simulink model "model_compatible"  (Simulink 7.5)
(part 2 of 2)

  bus83 : powerlib/Measurements/Load Flow Bus  LConnTagsString=a  Phases=single  Connectors=on one side  ID=bus83  Vbase=220000  Vref=1  Vangle=0  VLF=1  VLFb=1  VLFc=1  angleLF=0  angleLFb=0  angleLFc=0
      settings: AttributesFormatString=|
      | %<ID>
      | %<Vbase>V
      | %<VLF>pu
      | %<angleLF>deg.
      | %<Name>
  bus84 : powerlib/Measurements/Load Flow Bus  LConnTagsString=a  Phases=single  Connectors=on one side  ID=bus84  Vbase=220000  Vref=1  Vangle=0  VLF=1  VLFb=1  VLFc=1  angleLF=0  angleLFb=0  angleLFc=0
      settings: AttributesFormatString=|
      | %<ID>
      | %<Vbase>V
      | %<VLF>pu
      | %<angleLF>deg.
      | %<Name>
  bus85 : powerlib/Measurements/Load Flow Bus  LConnTagsString=a  Phases=single  Connectors=on one side  ID=bus85  Vbase=220000  Vref=1  Vangle=0  VLF=1  VLFb=1  VLFc=1  angleLF=0  angleLFb=0  angleLFc=0
      settings: AttributesFormatString=|
      | %<ID>
      | %<Vbase>V
      | %<VLF>pu
      | %<angleLF>deg.
      | %<Name>
  bus86 : powerlib/Measurements/Load Flow Bus  LConnTagsString=a  Phases=single  Connectors=on one side  ID=bus86  Vbase=220000  Vref=1  Vangle=0  VLF=1  VLFb=1  VLFc=1  angleLF=0  angleLFb=0  angleLFc=0
      settings: AttributesFormatString=|
      | %<ID>
      | %<Vbase>V
      | %<VLF>pu
      | %<angleLF>deg.
      | %<Name>
  bus87 : powerlib/Measurements/Load Flow Bus  LConnTagsString=a  Phases=single  Connectors=on one side  ID=bus87  Vbase=220000  Vref=1  Vangle=0  VLF=1  VLFb=1  VLFc=1  angleLF=0  angleLFb=0  angleLFc=0
      settings: AttributesFormatString=|
      | %<ID>
      | %<Vbase>V
      | %<VLF>pu
      | %<angleLF>deg.
      | %<Name>
  bus88 : powerlib/Measurements/Load Flow Bus  LConnTagsString=a  Phases=single  Connectors=on one side  ID=bus88  Vbase=220000  Vref=1  Vangle=0  VLF=1  VLFb=1  VLFc=1  angleLF=0  angleLFb=0  angleLFc=0
      settings: AttributesFormatString=|
      | %<ID>
      | %<Vbase>V
      | %<VLF>pu
      | %<angleLF>deg.
      | %<Name>
  bus89 : powerlib/Measurements/Load Flow Bus  LConnTagsString=a  Phases=single  Connectors=on one side  ID=bus89  Vbase=220000  Vref=1  Vangle=0  VLF=1  VLFb=1  VLFc=1  angleLF=0  angleLFb=0  angleLFc=0
      settings: AttributesFormatString=|
      | %<ID>
      | %<Vbase>V
      | %<VLF>pu
      | %<angleLF>deg.
      | %<Name>
  bus9 : powerlib/Measurements/Load Flow Bus  LConnTagsString=a  Phases=single  Connectors=on one side  ID=bus9  Vbase=220000  Vref=1  Vangle=0  VLF=1  VLFb=1  VLFc=1  angleLF=0  angleLFb=0  angleLFc=0
      settings: AttributesFormatString=|
      | %<ID>
      | %<Vbase>V
      | %<VLF>pu
      | %<angleLF>deg.
      | %<Name>
  bus90 : powerlib/Measurements/Load Flow Bus  LConnTagsString=a  Phases=single  Connectors=on one side  ID=bus90  Vbase=220000  Vref=1  Vangle=0  VLF=1  VLFb=1  VLFc=1  angleLF=0  angleLFb=0  angleLFc=0
      settings: AttributesFormatString=|
      | %<ID>
      | %<Vbase>V
      | %<VLF>pu
      | %<angleLF>deg.
      | %<Name>
  bus91 : powerlib/Measurements/Load Flow Bus  LConnTagsString=a  Phases=single  Connectors=on one side  ID=bus91  Vbase=220000  Vref=1  Vangle=0  VLF=1  VLFb=1  VLFc=1  angleLF=0  angleLFb=0  angleLFc=0
      settings: AttributesFormatString=|
      | %<ID>
      | %<Vbase>V
      | %<VLF>pu
      | %<angleLF>deg.
      | %<Name>
  bus92 : powerlib/Measurements/Load Flow Bus  LConnTagsString=a  Phases=single  Connectors=on one side  ID=bus92  Vbase=220000  Vref=1  Vangle=0  VLF=1  VLFb=1  VLFc=1  angleLF=0  angleLFb=0  angleLFc=0
      settings: AttributesFormatString=|
      | %<ID>
      | %<Vbase>V
      | %<VLF>pu
      | %<angleLF>deg.
      | %<Name>
  bus93 : powerlib/Measurements/Load Flow Bus  LConnTagsString=a  Phases=single  Connectors=on one side  ID=bus93  Vbase=220000  Vref=1  Vangle=0  VLF=1  VLFb=1  VLFc=1  angleLF=0  angleLFb=0  angleLFc=0
      settings: AttributesFormatString=|
      | %<ID>
      | %<Vbase>V
      | %<VLF>pu
      | %<angleLF>deg.
      | %<Name>
  bus94 : powerlib/Measurements/Load Flow Bus  LConnTagsString=a  Phases=single  Connectors=on one side  ID=bus94  Vbase=220000  Vref=1  Vangle=0  VLF=1  VLFb=1  VLFc=1  angleLF=0  angleLFb=0  angleLFc=0
      settings: AttributesFormatString=|
      | %<ID>
      | %<Vbase>V
      | %<VLF>pu
      | %<angleLF>deg.
      | %<Name>
  bus95 : powerlib/Measurements/Load Flow Bus  LConnTagsString=a  Phases=single  Connectors=on one side  ID=bus95  Vbase=220000  Vref=1  Vangle=0  VLF=1  VLFb=1  VLFc=1  angleLF=0  angleLFb=0  angleLFc=0
      settings: AttributesFormatString=|
      | %<ID>
      | %<Vbase>V
      | %<VLF>pu
      | %<angleLF>deg.
      | %<Name>
  bus96 : powerlib/Measurements/Load Flow Bus  LConnTagsString=a  Phases=single  Connectors=on one side  ID=bus96  Vbase=220000  Vref=1  Vangle=0  VLF=1  VLFb=1  VLFc=1  angleLF=0  angleLFb=0  angleLFc=0
      settings: AttributesFormatString=|
      | %<ID>
      | %<Vbase>V
      | %<VLF>pu
      | %<angleLF>deg.
      | %<Name>
  bus97 : powerlib/Measurements/Load Flow Bus  LConnTagsString=a  Phases=single  Connectors=on one side  ID=bus97  Vbase=220000  Vref=1  Vangle=0  VLF=1  VLFb=1  VLFc=1  angleLF=0  angleLFb=0  angleLFc=0
      settings: AttributesFormatString=|
      | %<ID>
      | %<Vbase>V
      | %<VLF>pu
      | %<angleLF>deg.
      | %<Name>
  bus98 : powerlib/Measurements/Load Flow Bus  LConnTagsString=a  Phases=single  Connectors=on one side  ID=bus98  Vbase=220000  Vref=1  Vangle=0  VLF=1  VLFb=1  VLFc=1  angleLF=0  angleLFb=0  angleLFc=0
      settings: AttributesFormatString=|
      | %<ID>
      | %<Vbase>V
      | %<VLF>pu
      | %<angleLF>deg.
      | %<Name>
  bus99 : powerlib/Measurements/Load Flow Bus  LConnTagsString=a  Phases=single  Connectors=on one side  ID=bus99  Vbase=220000  Vref=1  Vangle=0  VLF=1  VLFb=1  VLFc=1  angleLF=0  angleLFb=0  angleLFc=0
      settings: AttributesFormatString=|
      | %<ID>
      | %<Vbase>V
      | %<VLF>pu
      | %<angleLF>deg.
      | %<Name>
  powergui : powerlib/powergui  Priority=1  SimulationMode=Phasor  SolverType=Tustin/Backward Euler (TBE)  SampleTime=50e-6  frequency=50  SPID=off  DisableSnubberDevices=off  DisableRonSwitches=off  DisableVfSwitches=off  SwTol=0  DisplayEquations=off  Interpol=off  ExternalGateDelay=off  methode=off  Ts=10  FunctionMessages=off  echomessages=off  HookPort=off  EnableUseOfTLC=off  x0status=blocks  frequencyindice=50  Pbase=3000e6  ErrMax=0.0001  Iterations=50  UnitsV=V  UnitsW=W  buscounter=0  RestoreLinks=warning  ResistiveCurrentMeasurement=off  Frange=[0:2:500]  Ylog=off  Xlog=on  ShowGrid=off  save=off  variable=ZData  structure=0  ZoomFFT=off  StartTime=0.0  cycles=1  DisplayStyle=1  fundamental=60  FreqAxis=off  MaxFrequency=1000  frequencyindicesteady=1  RmsSteady=1  display=off
  connections:
  T_174347010_220000_Centrale_Electrique_de_Oued_Sly/LConn1 -- _CN_174347010_220000_CN_173670736_220000/LConn1
  T_174347010_220000_Centrale_Electrique_de_Oued_Sly/LConn2 -- _CN_174347010_220000_CN_173670736_220000/LConn2
  _CN_174347010_220000_CN_173670736_220000/LConn3 -- T_174347010_220000_Centrale_Electrique_de_Oued_Sly/LConn3 -- bus1/LConn1
  _CN_174347010_220000_CN_173670736_220000/RConn1 -- T_173670736_220000_Poste_électrique_de_Khemis_Miliana/LConn1 -- _CN_375972637_220000_CN_173670736_220000/LConn1
  _CN_174347010_220000_CN_173670736_220000/RConn2 -- T_173670736_220000_Poste_électrique_de_Khemis_Miliana/LConn2 -- _CN_375972637_220000_CN_173670736_220000/LConn2
  _CN_174347010_220000_CN_173670736_220000/RConn3 -- T_173670736_220000_Poste_électrique_de_Khemis_Miliana/LConn3 -- _CN_375972637_220000_CN_173670736_220000/LConn3 -- bus2/LConn1
  _CN_177004931_220000_CN_173534563_220000/LConn1 -- T_177004931__Poste_électrique_de_Chefia/RConn1 -- _CN_177004931_220000_CN_177004925_220000/LConn1 -- L_177004931/LConn1
  _CN_177004931_220000_CN_173534563_220000/LConn2 -- T_177004931__Poste_électrique_de_Chefia/RConn2 -- _CN_177004931_220000_CN_177004925_220000/LConn2 -- L_177004931/LConn2
  _CN_177004931_220000_CN_173534563_220000/LConn3 -- T_177004931__Poste_électrique_de_Chefia/RConn3 -- _CN_177004931_220000_CN_177004925_220000/LConn3 -- L_177004931/LConn3 -- bus3/LConn1
  _CN_177004931_220000_CN_173534563_220000/RConn1 -- T_173534563_220000_/LConn1 -- _CN_173534563_220000_CN_177004925_220000/LConn1 -- _CN_173534563_220000_CN_176932212_220000/LConn1
  _CN_177004931_220000_CN_173534563_220000/RConn2 -- T_173534563_220000_/LConn2 -- _CN_173534563_220000_CN_177004925_220000/LConn2 -- _CN_173534563_220000_CN_176932212_220000/LConn2
  _CN_177004931_220000_CN_173534563_220000/RConn3 -- T_173534563_220000_/LConn3 -- _CN_173534563_220000_CN_177004925_220000/LConn3 -- _CN_173534563_220000_CN_176932212_220000/LConn3 -- bus4/LConn1
  _CN_177004931_220000_CN_177004925_220000/RConn1 -- T_177004925__/LConn1 -- _CN_173534563_220000_CN_177004925_220000/RConn1
  _CN_177004931_220000_CN_177004925_220000/RConn2 -- T_177004925__/LConn2 -- _CN_173534563_220000_CN_177004925_220000/RConn2
  _CN_177004931_220000_CN_177004925_220000/RConn3 -- T_177004925__/LConn3 -- _CN_173534563_220000_CN_177004925_220000/RConn3 -- bus5/LConn1
  _CN_295277014_220000_CN_174419698_220000/LConn1 -- T_295277014_220000_/LConn1 -- _CN_295277014_220000_CN_176684982_220000/LConn1
  _CN_295277014_220000_CN_174419698_220000/LConn2 -- T_295277014_220000_/LConn2 -- _CN_295277014_220000_CN_176684982_220000/LConn2
  _CN_295277014_220000_CN_174419698_220000/LConn3 -- T_295277014_220000_/LConn3 -- _CN_295277014_220000_CN_176684982_220000/LConn3 -- bus6/LConn1
  _CN_295277014_220000_CN_174419698_220000/RConn1 -- T_174419698__/LConn1 -- _CN_174512806_220000_CN_174419698_220000/LConn1 -- _CN_174512286_220000_CN_174419698_220000/LConn1
  _CN_295277014_220000_CN_174419698_220000/RConn2 -- T_174419698__/LConn2 -- _CN_174512806_220000_CN_174419698_220000/LConn2 -- _CN_174512286_220000_CN_174419698_220000/LConn2
  _CN_295277014_220000_CN_174419698_220000/RConn3 -- T_174419698__/LConn3 -- _CN_174512806_220000_CN_174419698_220000/LConn3 -- bus7/LConn1 -- _CN_174512286_220000_CN_174419698_220000/LConn3
  _CN_295277014_220000_CN_176684982_220000/RConn1 -- T_176684982_220000_/LConn1 -- _CN_176684982_220000_CN_226914785_220000/LConn1 -- _CN_176684982_220000_CN_175343993_220000/LConn1
  _CN_295277014_220000_CN_176684982_220000/RConn2 -- T_176684982_220000_/LConn2 -- _CN_176684982_220000_CN_226914785_220000/LConn2 -- _CN_176684982_220000_CN_175343993_220000/LConn2
  _CN_295277014_220000_CN_176684982_220000/RConn3 -- T_176684982_220000_/LConn3 -- _CN_176684982_220000_CN_226914785_220000/LConn3 -- _CN_176684982_220000_CN_175343993_220000/LConn3 -- bus8/LConn1
  _CN_218114438_220000_CN_217976993_220000/LConn1 -- T_218114438__Centrale_Electrique/LConn1 -- _CN_218114438_220000_CN_364421786_220000/LConn1
  _CN_218114438_220000_CN_217976993_220000/LConn2 -- T_218114438__Centrale_Electrique/LConn2 -- _CN_218114438_220000_CN_364421786_220000/LConn2
  _CN_218114438_220000_CN_217976993_220000/LConn3 -- T_218114438__Centrale_Electrique/LConn3 -- _CN_218114438_220000_CN_364421786_220000/LConn3 -- bus9/LConn1
  _CN_218114438_220000_CN_217976993_220000/RConn1 -- T_217976993__/LConn1 -- _CN_217970970_220000_CN_217976993_220000/LConn1 -- _CN_217976993_220000_CN_217926709_220000/LConn1
  _CN_218114438_220000_CN_217976993_220000/RConn2 -- T_217976993__/LConn2 -- _CN_217970970_220000_CN_217976993_220000/LConn2 -- _CN_217976993_220000_CN_217926709_220000/LConn2
  _CN_218114438_220000_CN_217976993_220000/RConn3 -- T_217976993__/LConn3 -- _CN_217970970_220000_CN_217976993_220000/LConn3 -- _CN_217976993_220000_CN_217926709_220000/LConn3 -- bus10/LConn1
  _CN_218114438_220000_CN_364421786_220000/RConn1 -- G_364421786_/RConn1 -- _CN_217941443_220000_CN_364421786_220000/LConn1
  _CN_218114438_220000_CN_364421786_220000/RConn2 -- G_364421786_/RConn2 -- _CN_217941443_220000_CN_364421786_220000/LConn2
  _CN_218114438_220000_CN_364421786_220000/RConn3 -- G_364421786_/RConn3 -- _CN_217941443_220000_CN_364421786_220000/LConn3 -- bus11/LConn1
  _CN_93235592_220000_CN_143736898_220000/LConn1 -- T_93235592_220000_SONELGAZ/LConn1 -- _CN_93235592_220000_CN_380986745_220000/LConn1
  _CN_93235592_220000_CN_143736898_220000/LConn2 -- T_93235592_220000_SONELGAZ/LConn2 -- _CN_93235592_220000_CN_380986745_220000/LConn2
  _CN_93235592_220000_CN_143736898_220000/LConn3 -- T_93235592_220000_SONELGAZ/LConn3 -- _CN_93235592_220000_CN_380986745_220000/LConn3 -- bus12/LConn1
  _CN_93235592_220000_CN_143736898_220000/RConn1 -- T_143736898__/LConn1 -- _CN_143736898_220000_CN_173808767_220000/LConn1 -- _CN_143736898_220000_CN_380986745_220000/LConn1
  _CN_93235592_220000_CN_143736898_220000/RConn2 -- T_143736898__/LConn2 -- _CN_143736898_220000_CN_173808767_220000/LConn2 -- _CN_143736898_220000_CN_380986745_220000/LConn2
  _CN_93235592_220000_CN_143736898_220000/RConn3 -- T_143736898__/LConn3 -- _CN_143736898_220000_CN_173808767_220000/LConn3 -- _CN_143736898_220000_CN_380986745_220000/LConn3 -- bus13/LConn1
  _CN_93235592_220000_CN_380986745_220000/RConn1 -- T_380986745__/LConn1 -- _CN_143736898_220000_CN_380986745_220000/RConn1
  _CN_93235592_220000_CN_380986745_220000/RConn2 -- T_380986745__/LConn2 -- _CN_143736898_220000_CN_380986745_220000/RConn2
  _CN_93235592_220000_CN_380986745_220000/RConn3 -- T_380986745__/LConn3 -- _CN_143736898_220000_CN_380986745_220000/RConn3 -- bus14/LConn1
  T_177011339__Centre_de_Transformation_éléctrique_Hammadi_Krouma/LConn1 -- _CN_177011339_220000_CN_176932212_220000/LConn1
  T_177011339__Centre_de_Transformation_éléctrique_Hammadi_Krouma/LConn2 -- _CN_177011339_220000_CN_176932212_220000/LConn2
  _CN_177011339_220000_CN_176932212_220000/LConn3 -- T_177011339__Centre_de_Transformation_éléctrique_Hammadi_Krouma/LConn3 -- bus15/LConn1
  _CN_177011339_220000_CN_176932212_220000/RConn1 -- T_176932212__/RConn1 -- _CN_173534563_220000_CN_176932212_220000/RConn1 -- L_176932212/LConn1
  _CN_177011339_220000_CN_176932212_220000/RConn2 -- T_176932212__/RConn2 -- _CN_173534563_220000_CN_176932212_220000/RConn2 -- L_176932212/LConn2
  _CN_177011339_220000_CN_176932212_220000/RConn3 -- T_176932212__/RConn3 -- _CN_173534563_220000_CN_176932212_220000/RConn3 -- L_176932212/LConn3 -- bus16/LConn1
  T_365883660__Poste_électrique/LConn1 -- _CN_365883660_220000_CN_175343993_220000/LConn1
  T_365883660__Poste_électrique/LConn2 -- _CN_365883660_220000_CN_175343993_220000/LConn2
  _CN_365883660_220000_CN_175343993_220000/LConn3 -- T_365883660__Poste_électrique/LConn3 -- bus17/LConn1
  _CN_365883660_220000_CN_175343993_220000/RConn1 -- T_175343993__/LConn1 -- _CN_312609390_220000_CN_175343993_220000/LConn1 -- _CN_174512286_220000_CN_175343993_220000/LConn1 -- _CN_176684982_220000_CN_175343993_220000/RConn1 -- _CN_175176155_220000_CN_175343993_220000/LConn1
  _CN_365883660_220000_CN_175343993_220000/RConn2 -- T_175343993__/LConn2 -- _CN_312609390_220000_CN_175343993_220000/LConn2 -- _CN_174512286_220000_CN_175343993_220000/LConn2 -- _CN_176684982_220000_CN_175343993_220000/RConn2 -- _CN_175176155_220000_CN_175343993_220000/LConn2
  _CN_365883660_220000_CN_175343993_220000/RConn3 -- T_175343993__/LConn3 -- _CN_312609390_220000_CN_175343993_220000/LConn3 -- bus18/LConn1 -- _CN_174512286_220000_CN_175343993_220000/LConn3 -- _CN_176684982_220000_CN_175343993_220000/RConn3 -- _CN_175176155_220000_CN_175343993_220000/LConn3
  T_371240205__/LConn1 -- _CN_371240205_220000_CN_173677993_220000/LConn1
  T_371240205__/LConn2 -- _CN_371240205_220000_CN_173677993_220000/LConn2
  _CN_371240205_220000_CN_173677993_220000/LConn3 -- T_371240205__/LConn3 -- bus19/LConn1
  _CN_371240205_220000_CN_173677993_220000/RConn1 -- T_173677993_220000_/RConn1 -- _CN_173677993_220000_CN_173985839_220000/LConn1 -- L_173677993/LConn1
  _CN_371240205_220000_CN_173677993_220000/RConn2 -- T_173677993_220000_/RConn2 -- _CN_173677993_220000_CN_173985839_220000/LConn2 -- L_173677993/LConn2
  _CN_371240205_220000_CN_173677993_220000/RConn3 -- T_173677993_220000_/RConn3 -- _CN_173677993_220000_CN_173985839_220000/LConn3 -- L_173677993/LConn3 -- bus20/LConn1
  T_227962923__/LConn1 -- _CN_227962923_220000_CN_226918874_220000/LConn1
  T_227962923__/LConn2 -- _CN_227962923_220000_CN_226918874_220000/LConn2
  _CN_227962923_220000_CN_226918874_220000/LConn3 -- T_227962923__/LConn3 -- bus21/LConn1
  _CN_227962923_220000_CN_226918874_220000/RConn1 -- G_226918874_TRANSFORMATEUR_HAUTE_TENSION/RConn1 -- _CN_292110924_220000_CN_226918874_220000/LConn1
  _CN_227962923_220000_CN_226918874_220000/RConn2 -- G_226918874_TRANSFORMATEUR_HAUTE_TENSION/RConn2 -- _CN_292110924_220000_CN_226918874_220000/LConn2
  _CN_227962923_220000_CN_226918874_220000/RConn3 -- G_226918874_TRANSFORMATEUR_HAUTE_TENSION/RConn3 -- _CN_292110924_220000_CN_226918874_220000/LConn3 -- bus22/LConn1
  T_217933343__SONELGAZ/LConn1 -- _CN_217933343_220000_CN_217926709_220000/LConn1
  T_217933343__SONELGAZ/LConn2 -- _CN_217933343_220000_CN_217926709_220000/LConn2
  _CN_217933343_220000_CN_217926709_220000/LConn3 -- T_217933343__SONELGAZ/LConn3 -- bus23/LConn1
  _CN_217933343_220000_CN_217926709_220000/RConn1 -- G_217926709_Centrale_électrique_de_Hassi_Messaoud/RConn1 -- _CN_217976993_220000_CN_217926709_220000/RConn1 -- _CN_217933346_220000_CN_217926709_220000/LConn1 -- _CN_292487199_220000_CN_217926709_220000/LConn1 -- _CN_217926708_220000_CN_217926709_220000/LConn1 -- _CN_217926711_220000_CN_217926709_220000/LConn1
  _CN_217933343_220000_CN_217926709_220000/RConn2 -- G_217926709_Centrale_électrique_de_Hassi_Messaoud/RConn2 -- _CN_217976993_220000_CN_217926709_220000/RConn2 -- _CN_217933346_220000_CN_217926709_220000/LConn2 -- _CN_292487199_220000_CN_217926709_220000/LConn2 -- _CN_217926708_220000_CN_217926709_220000/LConn2 -- _CN_217926711_220000_CN_217926709_220000/LConn2
  _CN_217933343_220000_CN_217926709_220000/RConn3 -- G_217926709_Centrale_électrique_de_Hassi_Messaoud/RConn3 -- _CN_217976993_220000_CN_217926709_220000/RConn3 -- _CN_217933346_220000_CN_217926709_220000/LConn3 -- _CN_292487199_220000_CN_217926709_220000/LConn3 -- _CN_217926708_220000_CN_217926709_220000/LConn3 -- _CN_217926711_220000_CN_217926709_220000/LConn3 -- bus24/LConn1
  _CN_217970970_220000_CN_217976993_220000/RConn1 -- T_217970970_400000_/LConn1 -- _CN_217970970_220000_CN_217941443_220000/LConn1
  _CN_217970970_220000_CN_217976993_220000/RConn2 -- T_217970970_400000_/LConn2 -- _CN_217970970_220000_CN_217941443_220000/LConn2
  _CN_217970970_220000_CN_217976993_220000/RConn3 -- T_217970970_400000_/LConn3 -- _CN_217970970_220000_CN_217941443_220000/LConn3 -- bus25/LConn1
  _CN_217970970_220000_CN_217941443_220000/RConn1 -- T_217941443__/LConn1 -- _CN_217941443_220000_CN_364421786_220000/RConn1
  _CN_217970970_220000_CN_217941443_220000/RConn2 -- T_217941443__/LConn2 -- _CN_217941443_220000_CN_364421786_220000/RConn2
  _CN_217970970_220000_CN_217941443_220000/RConn3 -- T_217941443__/LConn3 -- _CN_217941443_220000_CN_364421786_220000/RConn3 -- bus26/LConn1
  T_107649691__Poste_électrique_Beni_Mered/LConn1 -- _CN_107649691_220000_CN_107619155_220000/LConn1
  T_107649691__Poste_électrique_Beni_Mered/LConn2 -- _CN_107649691_220000_CN_107619155_220000/LConn2
  _CN_107649691_220000_CN_107619155_220000/LConn3 -- T_107649691__Poste_électrique_Beni_Mered/LConn3 -- bus27/LConn1
  G_107619155_Centrale_électrique_de_Larbâa/RConn1 -- _CN_107649691_220000_CN_107619155_220000/RConn1
  G_107619155_Centrale_électrique_de_Larbâa/RConn2 -- _CN_107649691_220000_CN_107619155_220000/RConn2
  _CN_107649691_220000_CN_107619155_220000/RConn3 -- G_107619155_Centrale_électrique_de_Larbâa/RConn3 -- bus28/LConn1
  _CN_375972637_220000_CN_221085150_220000/LConn1 -- T_375972637__/LConn1 -- _CN_375972637_220000_CN_173670736_220000/RConn1 -- _CN_375972637_220000_CN_254853839_220000/LConn1
  _CN_375972637_220000_CN_221085150_220000/LConn2 -- T_375972637__/LConn2 -- _CN_375972637_220000_CN_173670736_220000/RConn2 -- _CN_375972637_220000_CN_254853839_220000/LConn2
  _CN_375972637_220000_CN_221085150_220000/LConn3 -- T_375972637__/LConn3 -- _CN_375972637_220000_CN_173670736_220000/RConn3 -- bus29/LConn1 -- _CN_375972637_220000_CN_254853839_220000/LConn3
  _CN_375972637_220000_CN_221085150_220000/RConn1 -- T_221085150_400000;220000_/RConn1 -- _CN_254853839_220000_CN_221085150_220000/LConn1 -- L_221085150/LConn1
  _CN_375972637_220000_CN_221085150_220000/RConn2 -- T_221085150_400000;220000_/RConn2 -- _CN_254853839_220000_CN_221085150_220000/LConn2 -- L_221085150/LConn2
  _CN_375972637_220000_CN_221085150_220000/RConn3 -- T_221085150_400000;220000_/RConn3 -- _CN_254853839_220000_CN_221085150_220000/LConn3 -- L_221085150/LConn3 -- bus30/LConn1
  _CN_375972637_220000_CN_254853839_220000/RConn1 -- T_254853839_220000_Sonelgaz/LConn1 -- _CN_254853839_220000_CN_221085150_220000/RConn1
  _CN_375972637_220000_CN_254853839_220000/RConn2 -- T_254853839_220000_Sonelgaz/LConn2 -- _CN_254853839_220000_CN_221085150_220000/RConn2
  _CN_375972637_220000_CN_254853839_220000/RConn3 -- T_254853839_220000_Sonelgaz/LConn3 -- _CN_254853839_220000_CN_221085150_220000/RConn3 -- bus31/LConn1
  _CN_174512286_220000_CN_175343993_220000/RConn1 -- T_174512286__Centrale_Electrique/RConn1 -- _CN_174512286_220000_CN_174419698_220000/RConn1 -- _CN_174512286_220000_CN_175299043_220000/LConn1 -- L_174512286/LConn1 -- _CN_174512286_220000_CN_175176155_220000/LConn1
  _CN_174512286_220000_CN_175343993_220000/RConn2 -- T_174512286__Centrale_Electrique/RConn2 -- _CN_174512286_220000_CN_174419698_220000/RConn2 -- _CN_174512286_220000_CN_175299043_220000/LConn2 -- L_174512286/LConn2 -- _CN_174512286_220000_CN_175176155_220000/LConn2
  _CN_174512286_220000_CN_175343993_220000/RConn3 -- T_174512286__Centrale_Electrique/RConn3 -- _CN_174512286_220000_CN_174419698_220000/RConn3 -- _CN_174512286_220000_CN_175299043_220000/LConn3 -- L_174512286/LConn3 -- bus32/LConn1 -- _CN_174512286_220000_CN_175176155_220000/LConn3
  _CN_174512286_220000_CN_175176155_220000/RConn1 -- T_175176155__/LConn1 -- _CN_175176155_220000_CN_175343993_220000/RConn1
  _CN_174512286_220000_CN_175176155_220000/RConn2 -- T_175176155__/LConn2 -- _CN_175176155_220000_CN_175343993_220000/RConn2
  _CN_174512286_220000_CN_175176155_220000/RConn3 -- T_175176155__/LConn3 -- _CN_175176155_220000_CN_175343993_220000/RConn3 -- bus33/LConn1
  T_175299043__/LConn1 -- _CN_174512286_220000_CN_175299043_220000/RConn1
  T_175299043__/LConn2 -- _CN_174512286_220000_CN_175299043_220000/RConn2
  _CN_174512286_220000_CN_175299043_220000/RConn3 -- T_175299043__/LConn3 -- bus34/LConn1
  T_107574175_220000_Station_Electrique_de_Boudouaou/LConn1 -- _CN_107574175_220000_CN_107644723_220000/LConn1
  T_107574175_220000_Station_Electrique_de_Boudouaou/LConn2 -- _CN_107574175_220000_CN_107644723_220000/LConn2
  _CN_107574175_220000_CN_107644723_220000/LConn3 -- T_107574175_220000_Station_Electrique_de_Boudouaou/LConn3 -- bus35/LConn1
  G_107644723_Centrale_électrique_de_Cap_Djinet/RConn1 -- _CN_107574175_220000_CN_107644723_220000/RConn1
  G_107644723_Centrale_électrique_de_Cap_Djinet/RConn2 -- _CN_107574175_220000_CN_107644723_220000/RConn2
  _CN_107574175_220000_CN_107644723_220000/RConn3 -- G_107644723_Centrale_électrique_de_Cap_Djinet/RConn3 -- bus36/LConn1
  T_217933346__/LConn1 -- _CN_217933346_220000_CN_217926709_220000/RConn1
  T_217933346__/LConn2 -- _CN_217933346_220000_CN_217926709_220000/RConn2
  _CN_217933346_220000_CN_217926709_220000/RConn3 -- T_217933346__/LConn3 -- bus37/LConn1
  T_174512806__/LConn1 -- _CN_174512806_220000_CN_174419698_220000/RConn1
  T_174512806__/LConn2 -- _CN_174512806_220000_CN_174419698_220000/RConn2
  _CN_174512806_220000_CN_174419698_220000/RConn3 -- T_174512806__/LConn3 -- bus38/LConn1
  _CN_173682343_220000_CN_294431650_220000/LConn1 -- T_173682343_400000_Centrale_électrique/RConn1 -- _CN_173682343_220000_CN_174338940_220000/LConn1 -- L_173682343/LConn1
  _CN_173682343_220000_CN_294431650_220000/LConn2 -- T_173682343_400000_Centrale_électrique/RConn2 -- _CN_173682343_220000_CN_174338940_220000/LConn2 -- L_173682343/LConn2
  _CN_173682343_220000_CN_294431650_220000/LConn3 -- T_173682343_400000_Centrale_électrique/RConn3 -- _CN_173682343_220000_CN_174338940_220000/LConn3 -- L_173682343/LConn3 -- bus39/LConn1
  _CN_173682343_220000_CN_294431650_220000/RConn1 -- T_294431650__/LConn1 -- _CN_294431650_220000_CN_226917743_220000/LConn1
  _CN_173682343_220000_CN_294431650_220000/RConn2 -- T_294431650__/LConn2 -- _CN_294431650_220000_CN_226917743_220000/LConn2
  _CN_173682343_220000_CN_294431650_220000/RConn3 -- T_294431650__/LConn3 -- _CN_294431650_220000_CN_226917743_220000/LConn3 -- bus40/LConn1
  T_174338940_220000_Poste_électrique/LConn1 -- _CN_173682343_220000_CN_174338940_220000/RConn1
  T_174338940_220000_Poste_électrique/LConn2 -- _CN_173682343_220000_CN_174338940_220000/RConn2
  _CN_173682343_220000_CN_174338940_220000/RConn3 -- T_174338940_220000_Poste_électrique/LConn3 -- bus41/LConn1
  _CN_292487199_220000_CN_217926709_220000/RConn1 -- T_292487199__/LConn1 -- _CN_292487199_220000_CN_217926710_220000/LConn1
  _CN_292487199_220000_CN_217926709_220000/RConn2 -- T_292487199__/LConn2 -- _CN_292487199_220000_CN_217926710_220000/LConn2
  _CN_292487199_220000_CN_217926709_220000/RConn3 -- T_292487199__/LConn3 -- _CN_292487199_220000_CN_217926710_220000/LConn3 -- bus42/LConn1
  T_217926710__/LConn1 -- _CN_292487199_220000_CN_217926710_220000/RConn1
  T_217926710__/LConn2 -- _CN_292487199_220000_CN_217926710_220000/RConn2
  _CN_292487199_220000_CN_217926710_220000/RConn3 -- T_217926710__/LConn3 -- bus43/LConn1
  G_173985839_Centrale_électrique_de_Bethioua/RConn1 -- _CN_173677993_220000_CN_173985839_220000/RConn1
  G_173985839_Centrale_électrique_de_Bethioua/RConn2 -- _CN_173677993_220000_CN_173985839_220000/RConn2
  _CN_173677993_220000_CN_173985839_220000/RConn3 -- G_173985839_Centrale_électrique_de_Bethioua/RConn3 -- bus44/LConn1
  T_226922540_220000_/LConn1 -- _CN_226922540_220000_CN_292110924_220000/LConn1
  T_226922540_220000_/LConn2 -- _CN_226922540_220000_CN_292110924_220000/LConn2
  _CN_226922540_220000_CN_292110924_220000/LConn3 -- T_226922540_220000_/LConn3 -- bus45/LConn1
  _CN_226922540_220000_CN_292110924_220000/RConn1 -- T_292110924_400000_/LConn1 -- _CN_292110924_220000_CN_226918874_220000/RConn1
  _CN_226922540_220000_CN_292110924_220000/RConn2 -- T_292110924_400000_/LConn2 -- _CN_292110924_220000_CN_226918874_220000/RConn2
  _CN_226922540_220000_CN_292110924_220000/RConn3 -- T_292110924_400000_/LConn3 -- _CN_292110924_220000_CN_226918874_220000/RConn3 -- bus46/LConn1
  _CN_226912498_220000_CN_312609390_220000/LConn1 -- T_226912498__/RConn1 -- L_226912498/LConn1
  _CN_226912498_220000_CN_312609390_220000/LConn2 -- T_226912498__/RConn2 -- L_226912498/LConn2
  _CN_226912498_220000_CN_312609390_220000/LConn3 -- T_226912498__/RConn3 -- L_226912498/LConn3 -- bus47/LConn1
  _CN_226912498_220000_CN_312609390_220000/RConn1 -- T_312609390__/LConn1 -- _CN_387845900_220000_CN_312609390_220000/LConn1 -- _CN_312609390_220000_CN_175343993_220000/RConn1
  _CN_226912498_220000_CN_312609390_220000/RConn2 -- T_312609390__/LConn2 -- _CN_387845900_220000_CN_312609390_220000/LConn2 -- _CN_312609390_220000_CN_175343993_220000/RConn2
  _CN_226912498_220000_CN_312609390_220000/RConn3 -- T_312609390__/LConn3 -- _CN_387845900_220000_CN_312609390_220000/LConn3 -- _CN_312609390_220000_CN_175343993_220000/RConn3 -- bus48/LConn1
  T_387693359__/LConn1 -- _CN_387693359_220000_CN_175176544_220000/LConn1
  T_387693359__/LConn2 -- _CN_387693359_220000_CN_175176544_220000/LConn2
  _CN_387693359_220000_CN_175176544_220000/LConn3 -- T_387693359__/LConn3 -- bus49/LConn1
  T_175176544__Centrale_électrique/LConn1 -- _CN_387693359_220000_CN_175176544_220000/RConn1
  T_175176544__Centrale_électrique/LConn2 -- _CN_387693359_220000_CN_175176544_220000/RConn2
  _CN_387693359_220000_CN_175176544_220000/RConn3 -- T_175176544__Centrale_électrique/LConn3 -- bus50/LConn1
  T_217926708__/LConn1 -- _CN_217926708_220000_CN_217926709_220000/RConn1
  T_217926708__/LConn2 -- _CN_217926708_220000_CN_217926709_220000/RConn2
  _CN_217926708_220000_CN_217926709_220000/RConn3 -- T_217926708__/LConn3 -- bus51/LConn1
  T_217926711__/LConn1 -- _CN_217926711_220000_CN_217926709_220000/RConn1
  T_217926711__/LConn2 -- _CN_217926711_220000_CN_217926709_220000/RConn2
  _CN_217926711_220000_CN_217926709_220000/RConn3 -- T_217926711__/LConn3 -- bus52/LConn1
  _CN_383755661_220000_CN_217930453_220000/LConn1 -- T_383755661__/LConn1 -- _CN_383755661_220000_CN_217930454_220000/LConn1
  _CN_383755661_220000_CN_217930453_220000/LConn2 -- T_383755661__/LConn2 -- _CN_383755661_220000_CN_217930454_220000/LConn2
  _CN_383755661_220000_CN_217930453_220000/LConn3 -- T_383755661__/LConn3 -- _CN_383755661_220000_CN_217930454_220000/LConn3 -- bus53/LConn1
  G_217930453_Sonelgaz_Hassi_Messaoud/RConn1 -- _CN_383755661_220000_CN_217930453_220000/RConn1
  G_217930453_Sonelgaz_Hassi_Messaoud/RConn2 -- _CN_383755661_220000_CN_217930453_220000/RConn2
  _CN_383755661_220000_CN_217930453_220000/RConn3 -- G_217930453_Sonelgaz_Hassi_Messaoud/RConn3 -- bus54/LConn1
  T_217930454__/LConn1 -- _CN_383755661_220000_CN_217930454_220000/RConn1
  T_217930454__/LConn2 -- _CN_383755661_220000_CN_217930454_220000/RConn2
  _CN_383755661_220000_CN_217930454_220000/RConn3 -- T_217930454__/LConn3 -- bus55/LConn1
  T_173808767_220000_Centrale_electrique/LConn1 -- _CN_143736898_220000_CN_173808767_220000/RConn1
  T_173808767_220000_Centrale_electrique/LConn2 -- _CN_143736898_220000_CN_173808767_220000/RConn2
  _CN_143736898_220000_CN_173808767_220000/RConn3 -- T_173808767_220000_Centrale_electrique/LConn3 -- bus56/LConn1
  G_226914785_Centrale_électrique_de_Jijel/RConn1 -- _CN_176684982_220000_CN_226914785_220000/RConn1
  G_226914785_Centrale_électrique_de_Jijel/RConn2 -- _CN_176684982_220000_CN_226914785_220000/RConn2
  _CN_176684982_220000_CN_226914785_220000/RConn3 -- G_226914785_Centrale_électrique_de_Jijel/RConn3 -- bus57/LConn1
  T_43843800__Poste_HT_de_Laghouat/LConn1 -- _CN_43843800_220000_CN_226985195_220000/LConn1
  T_43843800__Poste_HT_de_Laghouat/LConn2 -- _CN_43843800_220000_CN_226985195_220000/LConn2
  _CN_43843800_220000_CN_226985195_220000/LConn3 -- T_43843800__Poste_HT_de_Laghouat/LConn3 -- bus58/LConn1
  T_226985195_220000_/LConn1 -- _CN_43843800_220000_CN_226985195_220000/RConn1
  T_226985195_220000_/LConn2 -- _CN_43843800_220000_CN_226985195_220000/RConn2
  _CN_43843800_220000_CN_226985195_220000/RConn3 -- T_226985195_220000_/LConn3 -- bus59/LConn1
  T_226917743__/LConn1 -- _CN_294431650_220000_CN_226917743_220000/RConn1
  T_226917743__/LConn2 -- _CN_294431650_220000_CN_226917743_220000/RConn2
  _CN_294431650_220000_CN_226917743_220000/RConn3 -- T_226917743__/LConn3 -- bus60/LConn1
  T_387845900__/LConn1 -- _CN_387845900_220000_CN_312609390_220000/RConn1
  T_387845900__/LConn2 -- _CN_387845900_220000_CN_312609390_220000/RConn2
  _CN_387845900_220000_CN_312609390_220000/RConn3 -- T_387845900__/LConn3 -- bus61/LConn1
  _CN_177004931_400000_CN_255597927_400000/LConn1 -- T_177004931__Poste_électrique_de_Chefia/LConn1 -- _CN_177004931_400000_CN_176932212_400000/LConn1
  _CN_177004931_400000_CN_255597927_400000/LConn2 -- T_177004931__Poste_électrique_de_Chefia/LConn2 -- _CN_177004931_400000_CN_176932212_400000/LConn2
  _CN_177004931_400000_CN_255597927_400000/LConn3 -- T_177004931__Poste_électrique_de_Chefia/LConn3 -- _CN_177004931_400000_CN_176932212_400000/LConn3 -- bus62/LConn1
  G_255597927_Centrale_Electrique_de_Koudiet_Eddraouch/RConn1 -- _CN_177004931_400000_CN_255597927_400000/RConn1
  G_255597927_Centrale_Electrique_de_Koudiet_Eddraouch/RConn2 -- _CN_177004931_400000_CN_255597927_400000/RConn2
  _CN_177004931_400000_CN_255597927_400000/RConn3 -- G_255597927_Centrale_Electrique_de_Koudiet_Eddraouch/RConn3 -- bus63/LConn1
  _CN_177004931_400000_CN_176932212_400000/RConn1 -- T_176932212__/LConn1 -- _CN_176932212_400000_CN_174512286_400000/LConn1 -- _CN_176932212_400000_CN_176932210_400000/LConn1
  _CN_177004931_400000_CN_176932212_400000/RConn2 -- T_176932212__/LConn2 -- _CN_176932212_400000_CN_174512286_400000/LConn2 -- _CN_176932212_400000_CN_176932210_400000/LConn2
  _CN_177004931_400000_CN_176932212_400000/RConn3 -- T_176932212__/LConn3 -- _CN_176932212_400000_CN_174512286_400000/LConn3 -- _CN_176932212_400000_CN_176932210_400000/LConn3 -- bus64/LConn1
  T_173682343_400000_Centrale_électrique/LConn1 -- _CN_173682343_400000_CN_173677993_400000/LConn1
  T_173682343_400000_Centrale_électrique/LConn2 -- _CN_173682343_400000_CN_173677993_400000/LConn2
  _CN_173682343_400000_CN_173677993_400000/LConn3 -- T_173682343_400000_Centrale_électrique/LConn3 -- bus65/LConn1
  _CN_173682343_400000_CN_173677993_400000/RConn1 -- T_173677993_220000_/LConn1 -- _CN_173677993_400000_CN_173670759_400000/LConn1
  _CN_173682343_400000_CN_173677993_400000/RConn2 -- T_173677993_220000_/LConn2 -- _CN_173677993_400000_CN_173670759_400000/LConn2
  _CN_173682343_400000_CN_173677993_400000/RConn3 -- T_173677993_220000_/LConn3 -- _CN_173677993_400000_CN_173670759_400000/LConn3 -- bus66/LConn1
  _CN_173677993_400000_CN_173670759_400000/RConn1 -- T_173670759__Poste_électrique/LConn1 -- _CN_173670759_400000_CN_221085150_400000/LConn1 -- _CN_173670759_400000_CN_226673305_400000/LConn1 -- _CN_173670759_400000_CN_173680073_400000/LConn1
  _CN_173677993_400000_CN_173670759_400000/RConn2 -- T_173670759__Poste_électrique/LConn2 -- _CN_173670759_400000_CN_221085150_400000/LConn2 -- _CN_173670759_400000_CN_226673305_400000/LConn2 -- _CN_173670759_400000_CN_173680073_400000/LConn2
  _CN_173677993_400000_CN_173670759_400000/RConn3 -- T_173670759__Poste_électrique/LConn3 -- _CN_173670759_400000_CN_221085150_400000/LConn3 -- _CN_173670759_400000_CN_226673305_400000/LConn3 -- bus67/LConn1 -- _CN_173670759_400000_CN_173680073_400000/LConn3
  G_173680073_Centrale_électrique_Hadjret_Ennous/RConn1 -- _CN_173670759_400000_CN_173680073_400000/RConn1
  G_173680073_Centrale_électrique_Hadjret_Ennous/RConn2 -- _CN_173670759_400000_CN_173680073_400000/RConn2
  _CN_173670759_400000_CN_173680073_400000/RConn3 -- G_173680073_Centrale_électrique_Hadjret_Ennous/RConn3 -- bus68/LConn1
  _CN_173670759_400000_CN_221085150_400000/RConn1 -- T_221085150_400000;220000_/LConn1 -- _CN_226392269_400000_CN_221085150_400000/LConn1 -- _CN_221085150_400000_CN_226673305_400000/LConn1
  _CN_173670759_400000_CN_221085150_400000/RConn2 -- T_221085150_400000;220000_/LConn2 -- _CN_226392269_400000_CN_221085150_400000/LConn2 -- _CN_221085150_400000_CN_226673305_400000/LConn2
  _CN_173670759_400000_CN_221085150_400000/RConn3 -- T_221085150_400000;220000_/LConn3 -- _CN_226392269_400000_CN_221085150_400000/LConn3 -- _CN_221085150_400000_CN_226673305_400000/LConn3 -- bus69/LConn1
  _CN_173670759_400000_CN_226673305_400000/RConn1 -- T_226673305_400000_/LConn1 -- _CN_221085150_400000_CN_226673305_400000/RConn1
  _CN_173670759_400000_CN_226673305_400000/RConn2 -- T_226673305_400000_/LConn2 -- _CN_221085150_400000_CN_226673305_400000/RConn2
  _CN_173670759_400000_CN_226673305_400000/RConn3 -- T_226673305_400000_/LConn3 -- _CN_221085150_400000_CN_226673305_400000/RConn3 -- bus70/LConn1
  _CN_226392269_400000_CN_174512286_400000/LConn1 -- T_226392269__/LConn1 -- _CN_226392269_400000_CN_221085150_400000/RConn1
  _CN_226392269_400000_CN_174512286_400000/LConn2 -- T_226392269__/LConn2 -- _CN_226392269_400000_CN_221085150_400000/RConn2
  _CN_226392269_400000_CN_174512286_400000/LConn3 -- T_226392269__/LConn3 -- _CN_226392269_400000_CN_221085150_400000/RConn3 -- bus71/LConn1
  _CN_226392269_400000_CN_174512286_400000/RConn1 -- T_174512286__Centrale_Electrique/LConn1 -- _CN_226912498_400000_CN_174512286_400000/LConn1 -- _CN_176932212_400000_CN_174512286_400000/RConn1
  _CN_226392269_400000_CN_174512286_400000/RConn2 -- T_174512286__Centrale_Electrique/LConn2 -- _CN_226912498_400000_CN_174512286_400000/LConn2 -- _CN_176932212_400000_CN_174512286_400000/RConn2
  _CN_226392269_400000_CN_174512286_400000/RConn3 -- T_174512286__Centrale_Electrique/LConn3 -- _CN_226912498_400000_CN_174512286_400000/LConn3 -- _CN_176932212_400000_CN_174512286_400000/RConn3 -- bus72/LConn1
  T_226912498__/LConn1 -- _CN_226912498_400000_CN_174512286_400000/RConn1
  T_226912498__/LConn2 -- _CN_226912498_400000_CN_174512286_400000/RConn2
  _CN_226912498_400000_CN_174512286_400000/RConn3 -- T_226912498__/LConn3 -- bus73/LConn1
  G_176932210_Centrale_électrique_à_cycle_combiné_de_Skikda/RConn1 -- _CN_176932212_400000_CN_176932210_400000/RConn1
  G_176932210_Centrale_électrique_à_cycle_combiné_de_Skikda/RConn2 -- _CN_176932212_400000_CN_176932210_400000/RConn2
  _CN_176932212_400000_CN_176932210_400000/RConn3 -- G_176932210_Centrale_électrique_à_cycle_combiné_de_Skikda/RConn3 -- bus74/LConn1
  T_174347010_220000_Centrale_Electrique_de_Oued_Sly/RConn1 -- L_174347010/LConn1
  T_174347010_220000_Centrale_Electrique_de_Oued_Sly/RConn2 -- L_174347010/LConn2
  L_174347010/LConn3 -- T_174347010_220000_Centrale_Electrique_de_Oued_Sly/RConn3 -- bus75/LConn1
  T_173670736_220000_Poste_électrique_de_Khemis_Miliana/RConn1 -- L_173670736/LConn1
  T_173670736_220000_Poste_électrique_de_Khemis_Miliana/RConn2 -- L_173670736/LConn2
  L_173670736/LConn3 -- T_173670736_220000_Poste_électrique_de_Khemis_Miliana/RConn3 -- bus76/LConn1
  T_173534563_220000_/RConn1 -- L_173534563/LConn1
  T_173534563_220000_/RConn2 -- L_173534563/LConn2
  L_173534563/LConn3 -- T_173534563_220000_/RConn3 -- bus77/LConn1
  T_177004925__/RConn1 -- L_177004925/LConn1
  T_177004925__/RConn2 -- L_177004925/LConn2
  L_177004925/LConn3 -- T_177004925__/RConn3 -- bus78/LConn1
  T_295277014_220000_/RConn1 -- L_295277014/LConn1
  T_295277014_220000_/RConn2 -- L_295277014/LConn2
  L_295277014/LConn3 -- T_295277014_220000_/RConn3 -- bus79/LConn1
  T_174419698__/RConn1 -- L_174419698/LConn1
  T_174419698__/RConn2 -- L_174419698/LConn2
  L_174419698/LConn3 -- T_174419698__/RConn3 -- bus80/LConn1
  T_176684982_220000_/RConn1 -- L_176684982/LConn1
  T_176684982_220000_/RConn2 -- L_176684982/LConn2
  L_176684982/LConn3 -- T_176684982_220000_/RConn3 -- bus81/LConn1
  T_218114438__Centrale_Electrique/RConn1 -- L_218114438/LConn1
  T_218114438__Centrale_Electrique/RConn2 -- L_218114438/LConn2
  L_218114438/LConn3 -- T_218114438__Centrale_Electrique/RConn3 -- bus82/LConn1
  T_217976993__/RConn1 -- L_217976993/LConn1
  T_217976993__/RConn2 -- L_217976993/LConn2
  L_217976993/LConn3 -- T_217976993__/RConn3 -- bus83/LConn1
  T_93235592_220000_SONELGAZ/RConn1 -- L_93235592/LConn1
  T_93235592_220000_SONELGAZ/RConn2 -- L_93235592/LConn2
  L_93235592/LConn3 -- T_93235592_220000_SONELGAZ/RConn3 -- bus84/LConn1
  T_143736898__/RConn1 -- L_143736898/LConn1
  T_143736898__/RConn2 -- L_143736898/LConn2
  L_143736898/LConn3 -- T_143736898__/RConn3 -- bus85/LConn1
  T_380986745__/RConn1 -- L_380986745/LConn1
  T_380986745__/RConn2 -- L_380986745/LConn2
  L_380986745/LConn3 -- T_380986745__/RConn3 -- bus86/LConn1
  T_177011339__Centre_de_Transformation_éléctrique_Hammadi_Krouma/RConn1 -- L_177011339/LConn1
  T_177011339__Centre_de_Transformation_éléctrique_Hammadi_Krouma/RConn2 -- L_177011339/LConn2
  L_177011339/LConn3 -- T_177011339__Centre_de_Transformation_éléctrique_Hammadi_Krouma/RConn3 -- bus87/LConn1
  T_365883660__Poste_électrique/RConn1 -- L_365883660/LConn1
  T_365883660__Poste_électrique/RConn2 -- L_365883660/LConn2
  L_365883660/LConn3 -- T_365883660__Poste_électrique/RConn3 -- bus88/LConn1
  T_175343993__/RConn1 -- L_175343993/LConn1
  T_175343993__/RConn2 -- L_175343993/LConn2
  L_175343993/LConn3 -- T_175343993__/RConn3 -- bus89/LConn1
  T_371240205__/RConn1 -- L_371240205/LConn1
  T_371240205__/RConn2 -- L_371240205/LConn2
  L_371240205/LConn3 -- T_371240205__/RConn3 -- bus90/LConn1
  T_227962923__/RConn1 -- L_227962923/LConn1
  T_227962923__/RConn2 -- L_227962923/LConn2
  L_227962923/LConn3 -- T_227962923__/RConn3 -- bus91/LConn1
  T_217933343__SONELGAZ/RConn1 -- L_217933343/LConn1
  T_217933343__SONELGAZ/RConn2 -- L_217933343/LConn2
  L_217933343/LConn3 -- T_217933343__SONELGAZ/RConn3 -- bus92/LConn1
  T_217970970_400000_/RConn1 -- L_217970970/LConn1
  T_217970970_400000_/RConn2 -- L_217970970/LConn2
  L_217970970/LConn3 -- T_217970970_400000_/RConn3 -- bus93/LConn1
  T_217941443__/RConn1 -- L_217941443/LConn1
  T_217941443__/RConn2 -- L_217941443/LConn2
  L_217941443/LConn3 -- T_217941443__/RConn3 -- bus94/LConn1
  T_107649691__Poste_électrique_Beni_Mered/RConn1 -- L_107649691/LConn1
  T_107649691__Poste_électrique_Beni_Mered/RConn2 -- L_107649691/LConn2
  L_107649691/LConn3 -- T_107649691__Poste_électrique_Beni_Mered/RConn3 -- bus95/LConn1
  T_375972637__/RConn1 -- L_375972637/LConn1
  T_375972637__/RConn2 -- L_375972637/LConn2
  L_375972637/LConn3 -- T_375972637__/RConn3 -- bus96/LConn1
  T_254853839_220000_Sonelgaz/RConn1 -- L_254853839/LConn1
  T_254853839_220000_Sonelgaz/RConn2 -- L_254853839/LConn2
  L_254853839/LConn3 -- T_254853839_220000_Sonelgaz/RConn3 -- bus97/LConn1
  T_175176155__/RConn1 -- L_175176155/LConn1
  T_175176155__/RConn2 -- L_175176155/LConn2
  L_175176155/LConn3 -- T_175176155__/RConn3 -- bus98/LConn1
  T_175299043__/RConn1 -- L_175299043/LConn1
  T_175299043__/RConn2 -- L_175299043/LConn2
  L_175299043/LConn3 -- T_175299043__/RConn3 -- bus99/LConn1
  T_107574175_220000_Station_Electrique_de_Boudouaou/RConn1 -- L_107574175/LConn1
  T_107574175_220000_Station_Electrique_de_Boudouaou/RConn2 -- L_107574175/LConn2
  L_107574175/LConn3 -- T_107574175_220000_Station_Electrique_de_Boudouaou/RConn3 -- bus100/LConn1
  T_217933346__/RConn1 -- L_217933346/LConn1
  T_217933346__/RConn2 -- L_217933346/LConn2
  L_217933346/LConn3 -- T_217933346__/RConn3 -- bus101/LConn1
  T_174512806__/RConn1 -- L_174512806/LConn1
  T_174512806__/RConn2 -- L_174512806/LConn2
  L_174512806/LConn3 -- T_174512806__/RConn3 -- bus102/LConn1
  T_294431650__/RConn1 -- L_294431650/LConn1
  T_294431650__/RConn2 -- L_294431650/LConn2
  L_294431650/LConn3 -- T_294431650__/RConn3 -- bus103/LConn1
  T_174338940_220000_Poste_électrique/RConn1 -- L_174338940/LConn1
  T_174338940_220000_Poste_électrique/RConn2 -- L_174338940/LConn2
  L_174338940/LConn3 -- T_174338940_220000_Poste_électrique/RConn3 -- bus104/LConn1
  T_292487199__/RConn1 -- L_292487199/LConn1
  T_292487199__/RConn2 -- L_292487199/LConn2
  L_292487199/LConn3 -- T_292487199__/RConn3 -- bus105/LConn1
  T_217926710__/RConn1 -- L_217926710/LConn1
  T_217926710__/RConn2 -- L_217926710/LConn2
  L_217926710/LConn3 -- T_217926710__/RConn3 -- bus106/LConn1
  T_226922540_220000_/RConn1 -- L_226922540/LConn1
  T_226922540_220000_/RConn2 -- L_226922540/LConn2
  L_226922540/LConn3 -- T_226922540_220000_/RConn3 -- bus107/LConn1
  T_292110924_400000_/RConn1 -- L_292110924/LConn1
  T_292110924_400000_/RConn2 -- L_292110924/LConn2
  L_292110924/LConn3 -- T_292110924_400000_/RConn3 -- bus108/LConn1
  T_312609390__/RConn1 -- L_312609390/LConn1
  T_312609390__/RConn2 -- L_312609390/LConn2
  L_312609390/LConn3 -- T_312609390__/RConn3 -- bus109/LConn1
  T_387693359__/RConn1 -- L_387693359/LConn1
  T_387693359__/RConn2 -- L_387693359/LConn2
  L_387693359/LConn3 -- T_387693359__/RConn3 -- bus110/LConn1
  T_175176544__Centrale_électrique/RConn1 -- L_175176544/LConn1
  T_175176544__Centrale_électrique/RConn2 -- L_175176544/LConn2
  L_175176544/LConn3 -- T_175176544__Centrale_électrique/RConn3 -- bus111/LConn1
  T_217926708__/RConn1 -- L_217926708/LConn1
  T_217926708__/RConn2 -- L_217926708/LConn2
  L_217926708/LConn3 -- T_217926708__/RConn3 -- bus112/LConn1
  T_217926711__/RConn1 -- L_217926711/LConn1
  T_217926711__/RConn2 -- L_217926711/LConn2
  L_217926711/LConn3 -- T_217926711__/RConn3 -- bus113/LConn1
  T_383755661__/RConn1 -- L_383755661/LConn1
  T_383755661__/RConn2 -- L_383755661/LConn2
  L_383755661/LConn3 -- T_383755661__/RConn3 -- bus114/LConn1
  T_217930454__/RConn1 -- L_217930454/LConn1
  T_217930454__/RConn2 -- L_217930454/LConn2
  L_217930454/LConn3 -- T_217930454__/RConn3 -- bus115/LConn1
  T_173808767_220000_Centrale_electrique/RConn1 -- L_173808767/LConn1
  T_173808767_220000_Centrale_electrique/RConn2 -- L_173808767/LConn2
  L_173808767/LConn3 -- T_173808767_220000_Centrale_electrique/RConn3 -- bus116/LConn1
  T_43843800__Poste_HT_de_Laghouat/RConn1 -- L_43843800/LConn1
  T_43843800__Poste_HT_de_Laghouat/RConn2 -- L_43843800/LConn2
  L_43843800/LConn3 -- T_43843800__Poste_HT_de_Laghouat/RConn3 -- bus117/LConn1
  T_226985195_220000_/RConn1 -- L_226985195/LConn1
  T_226985195_220000_/RConn2 -- L_226985195/LConn2
  L_226985195/LConn3 -- T_226985195_220000_/RConn3 -- bus118/LConn1
  T_226917743__/RConn1 -- L_226917743/LConn1
  T_226917743__/RConn2 -- L_226917743/LConn2
  L_226917743/LConn3 -- T_226917743__/RConn3 -- bus119/LConn1
  T_387845900__/RConn1 -- L_387845900/LConn1
  T_387845900__/RConn2 -- L_387845900/LConn2
  L_387845900/LConn3 -- T_387845900__/RConn3 -- bus120/LConn1
  T_173670759__Poste_électrique/RConn1 -- L_173670759/LConn1
  T_173670759__Poste_électrique/RConn2 -- L_173670759/LConn2
  L_173670759/LConn3 -- T_173670759__Poste_électrique/RConn3 -- bus121/LConn1
  T_226673305_400000_/RConn1 -- L_226673305/LConn1
  T_226673305_400000_/RConn2 -- L_226673305/LConn2
  L_226673305/LConn3 -- T_226673305_400000_/RConn3 -- bus122/LConn1
  T_226392269__/RConn1 -- L_226392269/LConn1
  T_226392269__/RConn2 -- L_226392269/LConn2
  L_226392269/LConn3 -- T_226392269__/RConn3 -- bus123/LConn1
